simulink model "simulaz"  (R2018b)
settings: Solver=ode4  StartTime=0.0  StopTime=T_end  FixedStep=Ts/10  RelTol=1e-3
values from neighbouring files (symbols this model uses):
  speed_ref = u(1)    [simulink_traj.m]
  Td_max = m*1.7*0.303    (= 883.3965)    [Parameters.m]
  Td_min = -m*9.81*0.303    (= -5097.71745)    [Parameters.m]
  theta = [m;Jz;a;b;Cf;Cr;rw;mu;Af;Al;Cx;Rr;rho;g]    [Parameters.m]
  Ts = 0.1    [maincode.m]
  xi_0 = [X Y Ux beta psi r]'    [maincode.m]
undefined symbols (not defined in the file or in its folder): den_dyn, num_dyn, num_int
settings Model: Creator=edoz9  LastModifiedBy=edoz9
settings DataIOCC: SaveOutput=off  SignalLogging=off  DSMLogging=off

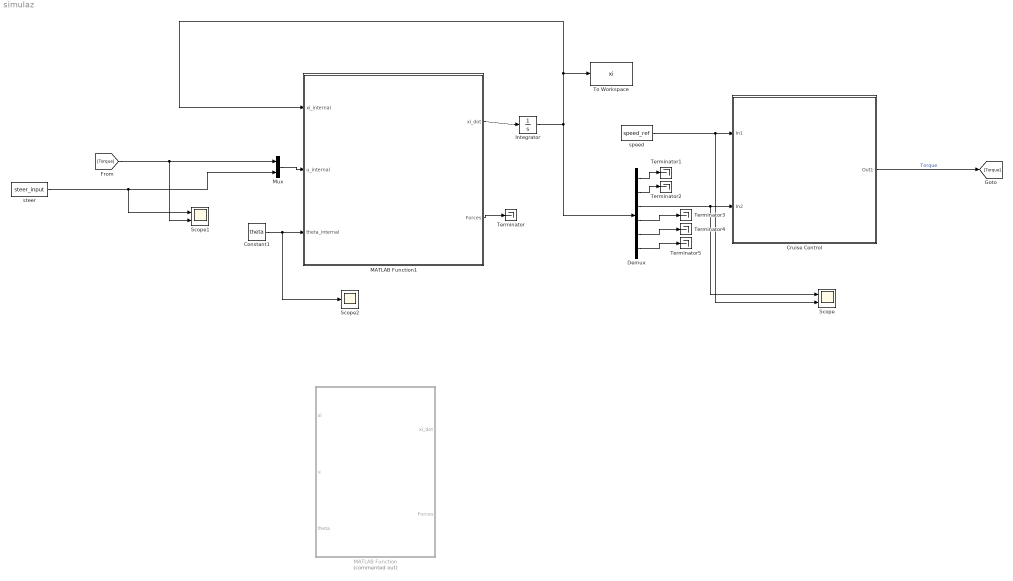
== system simulaz ==
  Constant1 : Constant  Value=theta
  Cruise Control : Subsystem
  Demux : Demux  Outputs=6
  Integrator : Integrator  InitialCondition=xi_0
  MATLAB Function : MATLAB Function  Commented=on  TreatAsAtomicUnit=on
  MATLAB Function1 : MATLAB Function  TreatAsAtomicUnit=on
  Mux : Mux  Inputs=2
  Scope : Scope  NumInputPorts=2
  Scope1 : Scope  NumInputPorts=2
  Scope2 : Scope
  Terminator{,1..5} (6 alike) : Terminator
  To Workspace : ToWorkspace  VariableName=xi  SaveFormat=Structure With Time  SampleTime=-1
      settings: Save2DSignal=2-D array (concatenate along first dimension)
  speed : Constant  Value=speed_ref
  steer : FromWorkspace  VariableName=steer_input  SampleTime=Ts  Interpolate=off  OutputAfterFinalValue=Setting to zero
  wires:
  steer/1 -> Scope1/1, Mux/2
  Cruise Control/1(Out1) -> [Torque]  "Torque"
  [Torque] -> Mux/1, Scope1/2
  speed/1 -> Scope/2, Cruise Control/1(In1)
  Demux/3 -> Scope/1, Cruise Control/2(In2)
  Demux/1 -> Terminator1/1
  Demux/2 -> Terminator2/1
  Demux/4 -> Terminator3/1
  Demux/5 -> Terminator4/1
  Demux/6 -> Terminator5/1
  Integrator/1 -> To Workspace/1, MATLAB Function1/1(xi_internal), Demux/1
  MATLAB Function1/1(xi_dot) -> Integrator/1
  Constant1/1 -> Scope2/1, MATLAB Function1/3(theta_internal)
  Mux/1 -> MATLAB Function1/2(u_internal)
  MATLAB Function1/2(Forces) -> Terminator/1

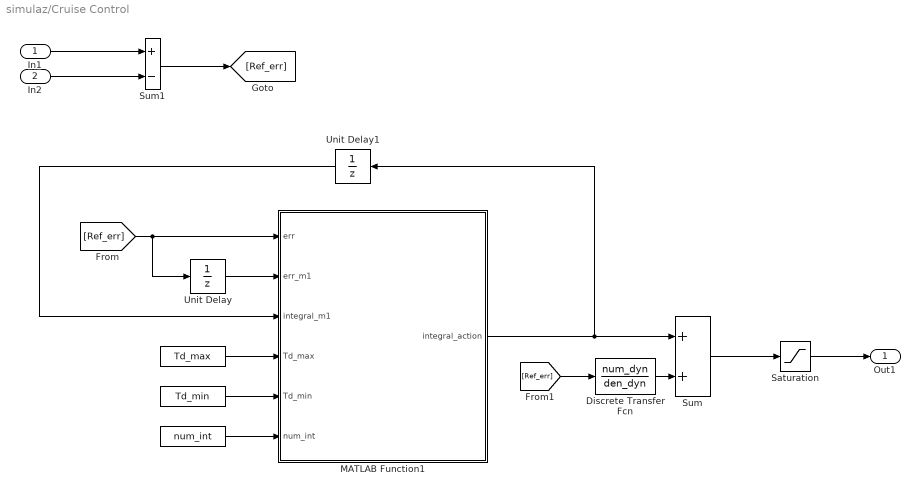
== system simulaz/Cruise Control ==
  In1 : Inport
  In2 : Inport  Port=2
  " " : Constant  Value=Td_min
  "  " : Constant  Value=num_int
  "   " : Constant  Value=Td_max
  Discrete Transfer Fcn : DiscreteTransferFcn  Numerator=num_dyn  Denominator=den_dyn
  MATLAB Function1 : MATLAB Function  TreatAsAtomicUnit=on
  Saturation : Saturate  UpperLimit=Td_max  LowerLimit=Td_min
  Sum : Sum
  Sum1 : Sum  Inputs=+-
  Unit Delay : UnitDelay  SampleTime=-1
  Unit Delay1 : UnitDelay  SampleTime=-1
  Out1 : Outport
  wires:
  " "/1 -> MATLAB Function1/5(Td_min)
  Unit Delay/1 -> MATLAB Function1/2(err_m1)
  [Ref_err] -> Unit Delay/1, MATLAB Function1/1(err)
  "   "/1 -> MATLAB Function1/4(Td_max)
  MATLAB Function1/1(integral_action) -> Sum/1, Unit Delay1/1
  Discrete Transfer Fcn/1 -> Sum/2
  Sum/1 -> Saturation/1
  In1/1 -> Sum1/1
  In2/1 -> Sum1/2
  Sum1/1 -> [Ref_err]
  [Ref_err] -> Discrete Transfer Fcn/1
  Saturation/1 -> Out1/1
  "  "/1 -> MATLAB Function1/6(num_int)
  Unit Delay1/1 -> MATLAB Function1/3(integral_m1)

== matlab function simulaz/Cruise Control/MATLAB Function1 ==
  data: err input; integral_action output; err_m1 input; integral_m1 input; Td_max input; Td_min input; num_int input
function integral_action = integrator_anti_wu(err, err_m1, integral_m1, Td_max, Td_min, num_int)

integral_action = min(Td_max, max(Td_min, integral_m1+num_int'*[err;err_m1]));

== matlab function simulaz/MATLAB Function ==
  data: xi input; u input; xi_dot output; theta input; Forces output
function [xi_dot,Forces] = Vehicle_Model_Function(xi,u,theta)
% Nonlinear dynamic model of a road vehicle with six states: 2-D position,
% 2-D velocity, yaw angle and yaw rate. Nonlinear lateral tyre forces with
% Fiala model; saturation on braking and driving torque, saturation on 
% front wheel steering angle. Partial de-coupling of longitudinal and
% lateral dynamics (assume longitudinal speed varies slowly with respect to
% lateral dynamics)
%
% Inputs:   tau     (time - for use with ode45)
%           xi      (model state)
%           u       (braking/driving torque and steering angle)
%           d       (lateral wind),
%           
%           theta   (model parameters)
%
% Outputs:  xi_dot  (derivative of the state with respect to time)
%           Forces  (longitudinal and lateral forces)

%% Read states

g = 9.81;

X       = xi(1,1);          % inertial X position (m)                 
Y       = xi(2,1);          % inertial Y position (m)
Ux      = xi(3,1);          % body x velocity (m/s)
beta    = xi(4,1);          % sideslip angle (rad)
psi     = xi(5,1);          % yaw angle (rad)
r       = xi(6,1);          % yaw rate (rad/s)

%% Read inputs
d = 0;
Td      = u(1,1);           % driving/braking torque (N*m)
delta   = u(2,1);           % front wheel steering angle (rad)
W       = d(1,1);           % lateral wind speed (m/s)

%% Parameter vector

m       = theta(1,1);       % vehicle mass (kg)
Jz      = theta(2,1);       % vehicle moment of inertia (kg*m^2)
a       = theta(3,1);       % distance between center of gravity and front axle (m)
b       = theta(4,1);       % distance between center of gravity and rear axle (m)
Cf      = theta(5,1);       % front axle cornering stiffness (N/rad)
Cr      = theta(6,1);       % rear axle cornering stiffness (N/rad)
rw      = theta(7,1);       % wheel radius (m)
mu      = theta(8,1);       % road friction coefficient
Af      = theta(9,1);       % vehicle front surface (m^2)
Al      = theta(10,1);      % vehicle lateral surface (m^2)
Cx      = theta(11,1);      % vehicle front aerodynamic drag coefficient
Rr      = theta(12,1);      % rolling resistance coefficient(N*s/m)
rho     = theta(13,1);      % air density (kg/m^3)


%% Equations

Uy      = tan( beta )*Ux;

% Tire slip angles
alphaf  = atan( (Uy + a*r)/(Ux) ) - delta;
alphar  = atan( (Uy - b*r)/(Ux) );

% Terms to compute the "FIALA MODEL"
zf      = tan(alphaf);
zr      = tan(alphar);

%% Forces

% Vertical Loads
Fzf     = m*g*( b/(a+b) );
Fzr     = m*g*( a/(a+b) );

% Lateral Forces
Fyf     = min( mu*Fzf, max( -mu*Fzf,-Cf*zf + ( Cf^2*abs(zf)*zf )/( 3*mu*Fzf ) - (Cf^3*zf^3)/(27*mu^2*Fzf^2) ) );
Fyr     = min( mu*Fzr, max( -mu*Fzr,-Cr*zr + ( Cr^2*abs(zr)*zr )/( 3*mu*Fzr ) - (Cr^3*zr^3)/(27*mu^2*Fzr^2) ) );

% Aerodynamic Lateral Force
Fyd     = (1/2)*rho*Al*W^2;

% Force acting along the local x direction (on the rear wheel)
Fx      = Td/rw;

% Rolling resistance Force
Fr      = Rr*Ux;

% Aerodynamic longitudinal Force
Fxd     = (1/2)*rho*Af*Cx*Ux^2;

%% State equations

X_dot        = Ux*cos(psi) - Uy*sin(psi);
Y_dot        = Ux*sin(psi) + Uy*cos(psi);
Ux_dot       = ( (Fx - Fyf*sin(delta)) - Fr - Fxd )/( m );
beta_dot     = ( Fyf*cos(delta) + Fyr + Fyd )/( m*Ux ) - r;
psi_dot      = r;
r_dot        = ( a*Fyf*cos(delta) - b*Fyr )/( Jz );

xi_dot = zeros(6,1);
xi_dot(1,1)  = X_dot;
xi_dot(2,1)  = Y_dot;
xi_dot(3,1)  = Ux_dot;
xi_dot(4,1)  = beta_dot;
xi_dot(5,1)  = psi_dot;
xi_dot(6,1)  = r_dot;

Forces = zeros(3,1);
Forces(1,1)  = Fyf; 
Forces(2,1)  = Fyr;
Forces(3,1)  = Fx;

end

== matlab function simulaz/MATLAB Function1 ==
  data: xi_internal input; u_internal input; xi_dot output; theta_internal input; Forces output
function [xi_dot, Forces] = vehicle(xi_internal, u_internal, theta_internal)
% simulation, time has to be the fist input

%% Read states
X = xi_internal(1,1);
Y = xi_internal(2,1);
Ux = xi_internal(3,1);
beta = xi_internal(4,1);
psi = xi_internal(5,1);
r = xi_internal(6,1);

%% Read Inputs

Td_internal = u_internal(1,1);
delta_internal = u_internal(2,1);

%% Read Parameters

m = theta_internal(1,1);
Jz = theta_internal(2,1);
a = theta_internal(3,1);
b = theta_internal(4,1);
Cf = theta_internal(5,1);
Cr = theta_internal(6,1);
rw = theta_internal(7,1);
mu = theta_internal(8,1);
Af = theta_internal(9,1);
Al = theta_internal(10,1);
Cx = theta_internal(11,1);
Rr = theta_internal(12,1);
rho = theta_internal(13,1);
g = theta_internal(14,1);

%% Equations

Uy = tan(beta)*Ux;
alfa_f = atan2((Uy + a*r),Ux) - delta_internal;
alfa_r = atan2((Uy - b*r),Ux);

F_z_f = m * g * b / (a+b);
F_z_r = m * g * a / (a+b);

z_f = tan(alfa_f);
z_r = tan(alfa_r);

elem1 = mu*F_z_f;
elem21 = - mu*F_z_f;
elem22 = - Cf*z_f + (Cf^2*abs(z_f)*z_f)/(3*mu*F_z_f) - (Cf^3*z_f^3)/(27*mu^2*F_z_f^2);
elem2 = max(elem21,elem22);
F_y_f = min(elem1, elem2);

elem1 = mu*F_z_r;
elem21 = - mu*F_z_r;
elem22 = - Cr*z_r + (Cr^2*abs(z_r)*z_r)/(3*mu*F_z_r) - (Cr^3*z_r^3)/(27*mu^2*F_z_r^2);
elem2 = max(elem21,elem22);
F_y_r = min(elem1,elem2);

F_x = Td_internal/rw;

F_r = Rr*Ux;
F_x_d = 0.5*rho*Af*Cx*Ux^2;

%% Output
xi_dot = zeros(6,1);
xi_dot(1,1) = Ux*cos(psi) - Uy*sin(psi);
xi_dot(2,1) = Ux*sin(psi)+ Uy*cos(psi);
xi_dot(3,1) = 1/m * ((F_x - F_y_f*sin(delta_internal))-F_r-F_x_d);
xi_dot(4,1) = 1/(m*Ux) * (F_y_f*cos(delta_internal)+F_y_r) - r;
xi_dot(5,1) = r;
xi_dot(6,1) = 1/Jz * (a*F_y_f*cos(delta_internal) - b* F_y_r);
Forces = zeros(3,1);
Forces(1,1) = F_y_f;
Forces(2,1) = F_y_r;
Forces(3,1) = F_x;

end
